simulink model "lab3termostat"  (R2013b)
settings: Solver=ode3  StartTime=0.0  StopTime=10.0  FixedStep=0.01  RelTol=1e-3
settings Model: Creator=User  LastModifiedBy=User

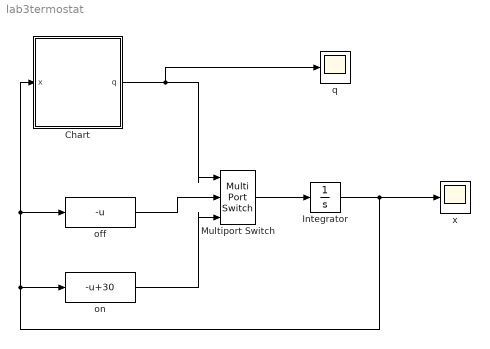
== system lab3termostat ==
  Chart : Stateflow chart  TreatAsAtomicUnit=on
  Integrator : Integrator
  Multiport Switch : MultiPortSwitch  Inputs=2
  off : MATLABFcn  MATLABFcn=-u  OutputSignalType=real
  on : MATLABFcn  MATLABFcn=-u+30  OutputSignalType=real
  q : Scope
  x : Scope
      settings: TimeRange=10
  wires:
  Multiport Switch/1 -> Integrator/1
  Integrator/1 -> x/1, on/1, off/1, Chart/1(x)
  off/1 -> Multiport Switch/2
  on/1 -> Multiport Switch/3
  Chart/1(q) -> Multiport Switch/1, q/1

== stateflow chart lab3termostat/Chart ==
  state off
    entry:q=1;
  state on
    entry:q=2;
  (default) -> off
  off -> on : [x<=19]
  on -> off : [x>=21]
  data: x input; q output double
